simulink model "climateCtrl"  (Simulink 8.0)
settings: Solver=VariableStepDiscrete  StartTime=0.0  StopTime=20  RelTol=1e-3
PreLoadFcn:
  | dT = 2;
libraries: simulink x1
settings Model: Creator=jrivitus  LastModifiedBy=ZhouHaoyu
settings DataIOCC: SignalLoggingSaveFormat=ModelDataLogs
settings OptimizationCC: EfficientMapNaN2IntZero=off
settings DebuggingCC: FcnCallInpInsideContextMsg=UseLocalSettings  StrictBusMsg=Warning
settings GRTTargetCC: CombineOutputUpdateFcns=off  GRTInterface=on

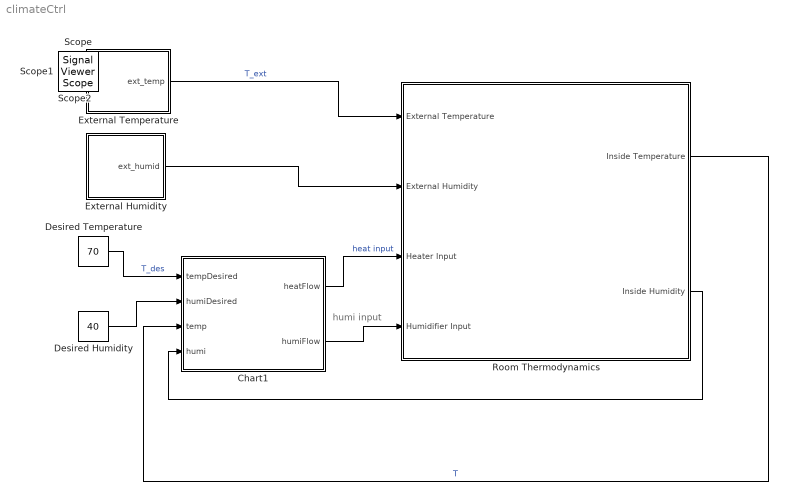
== system climateCtrl ==
  note: humi input
  Chart1 : Stateflow chart  TreatAsAtomicUnit=on
  Desired Humidity : Constant  Value=40
  Desired Temperature : Constant  Value=70
  External Humidity : Subsystem
  External Temperature : Subsystem
  Room Thermodynamics : Subsystem
  Scope : SignalViewerScope  IOType=viewer  RefreshTime=0.035000
      settings: TimeRange=20  YMin=50  YMax=100
  Scope1 : SignalViewerScope  IOType=viewer  RefreshTime=0.035000
  Scope2 : SignalViewerScope  IOType=viewer  RefreshTime=0.035000
      settings: SaveName=ScopeData2
  wires:
  External Temperature/1(ext_temp) -> Room Thermodynamics/1(External Temperature)  "T_ext"
  Chart1/1(heatFlow) -> Room Thermodynamics/3(Heater Input)  "heat input"
  Desired Temperature/1 -> Chart1/1(tempDesired)  "T_des"
  Room Thermodynamics/1(Inside Temperature) -> Chart1/3(temp)  "T"
  External Humidity/1(ext_humid) -> Room Thermodynamics/2(External Humidity)
  Room Thermodynamics/2(Inside Humidity) -> Chart1/4(humi)
  Desired Humidity/1 -> Chart1/2(humiDesired)
  Chart1/2(humiFlow) -> Room Thermodynamics/4(Humidifier Input)

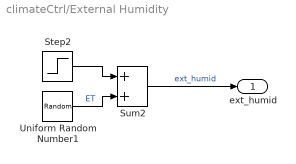
== system climateCtrl/External Humidity ==
  Step2 : Step  Time=10  Before=35  After=25  SampleTime=0.1
  Sum2 : Sum  SaturateOnIntegerOverflow=on
  Uniform Random Number1 : UniformRandomNumber  Minimum=-10  Maximum=10  SampleTime=0.1
  ext_humid : Outport
  wires:
  Sum2/1 -> ext_humid/1  "ext_humid"
  Step2/1 -> Sum2/1
  Uniform Random Number1/1 -> Sum2/2  "ET"

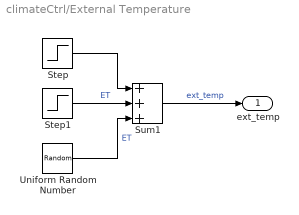
== system climateCtrl/External Temperature ==
  Step : Step  Time=15  Before=70  After=40  SampleTime=0.1
  Step1 : Step  Time=5  After=20  SampleTime=0.1
  Sum1 : Sum  Inputs=+++  SaturateOnIntegerOverflow=on
  Uniform Random Number : UniformRandomNumber  Minimum=-10  Maximum=10  SampleTime=0.1
  ext_temp : Outport
  wires:
  Step1/1 -> Sum1/2  "ET"
  Step/1 -> Sum1/1
  Uniform Random Number/1 -> Sum1/3  "ET"
  Sum1/1 -> ext_temp/1  "ext_temp"

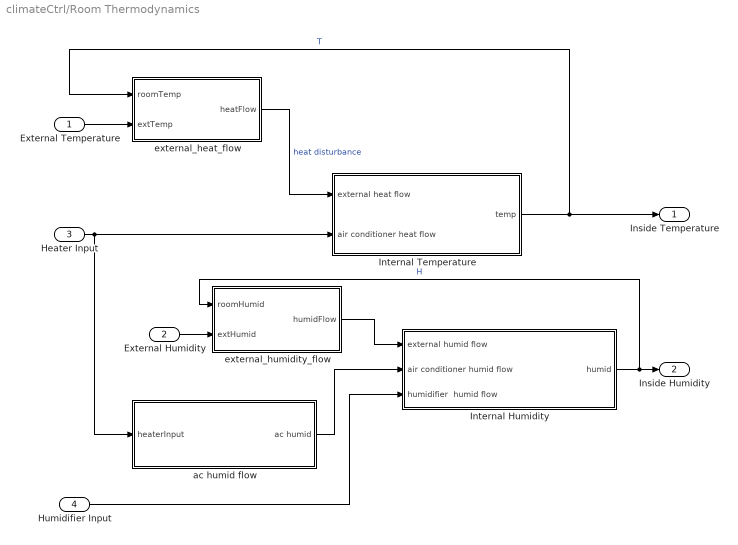
== system climateCtrl/Room Thermodynamics ==
  External Temperature : Inport
  External Humidity : Inport  Port=2
  Heater Input : Inport  Port=3
  Humidifier Input : Inport  Port=4
  Internal Humidity : Subsystem
  Internal Temperature : Subsystem
  ac humid flow : Subsystem
  external_heat_flow : Subsystem
  external_humidity_flow : Subsystem
  Inside Temperature : Outport
  Inside Humidity : Outport  Port=2
  wires:
  external_heat_flow/1(heatFlow) -> Internal Temperature/1(external heat flow)  "heat disturbance"
  Internal Temperature/1(temp) -> external_heat_flow/1(roomTemp), Inside Temperature/1  "T"
  External Temperature/1 -> external_heat_flow/2(extTemp)
  Heater Input/1 -> Internal Temperature/2(air conditioner heat flow), ac humid flow/1(heaterInput)
  External Humidity/1 -> external_humidity_flow/2(extHumid)
  external_humidity_flow/1(humidFlow) -> Internal Humidity/1(external humid flow)
  Internal Humidity/1(humid) -> external_humidity_flow/1(roomHumid), Inside Humidity/1  "H"
  Humidifier Input/1 -> Internal Humidity/3(humidifier  humid flow)
  ac humid flow/1(ac humid) -> Internal Humidity/2(air conditioner humid flow)

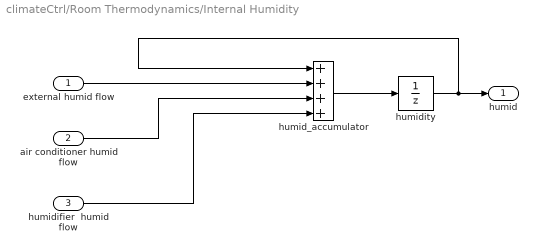
== system climateCtrl/Room Thermodynamics/Internal Humidity ==
  external humid flow : Inport
  air conditioner humid flow : Inport  Port=2
  humidifier  humid flow : Inport  Port=3
  humid_accumulator : Sum  Inputs=++++
  humidity : UnitDelay  InitialCondition=40  SampleTime=-1
  humid : Outport
  wires:
  air conditioner humid flow/1 -> humid_accumulator/3
  external humid flow/1 -> humid_accumulator/2
  humidity/1 -> humid_accumulator/1, humid/1
  humid_accumulator/1 -> humidity/1
  humidifier  humid flow/1 -> humid_accumulator/4

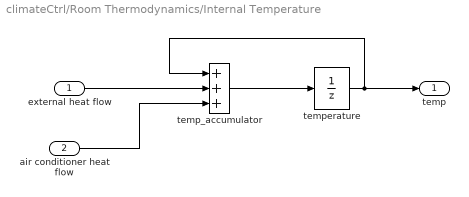
== system climateCtrl/Room Thermodynamics/Internal Temperature ==
  external heat flow : Inport
  air conditioner heat flow : Inport  Port=2
  temp_accumulator : Sum  Inputs=+++
  temperature : UnitDelay  InitialCondition=70  SampleTime=0.1
  temp : Outport
  wires:
  air conditioner heat flow/1 -> temp_accumulator/3
  external heat flow/1 -> temp_accumulator/2
  temp_accumulator/1 -> temperature/1
  temperature/1 -> temp/1, temp_accumulator/1

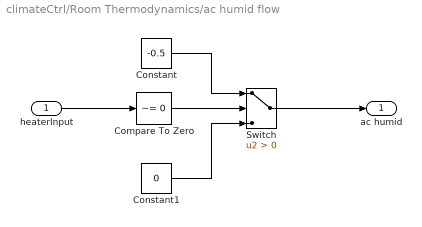
== system climateCtrl/Room Thermodynamics/ac humid flow ==
  heaterInput : Inport
  Compare To Zero : simulink/Logic and Bit Operations/Compare To Zero  relop=~=  OutDataTypeStr=uint8  ZeroCross=off
  Constant : Constant  Value=-0.5
  Constant1 : Constant  Value=0
  Switch : Switch  Criteria=u2 > Threshold
  ac humid : Outport  OutDataTypeStr=double  InitialOutput=0
  wires:
  heaterInput/1 -> Compare To Zero/1
  Compare To Zero/1 -> Switch/2
  Constant/1 -> Switch/1
  Constant1/1 -> Switch/3
  Switch/1 -> ac humid/1

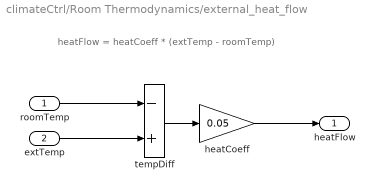
== system climateCtrl/Room Thermodynamics/external_heat_flow ==
  note: heatFlow = heatCoeff * (extTemp - roomTemp)
  roomTemp : Inport
  extTemp : Inport  Port=2
  heatCoeff : Gain  Gain=0.05
  tempDiff : Sum  Inputs=-+
  heatFlow : Outport  OutDataTypeStr=double  InitialOutput=0
  wires:
  extTemp/1 -> tempDiff/2
  roomTemp/1 -> tempDiff/1
  heatCoeff/1 -> heatFlow/1
  tempDiff/1 -> heatCoeff/1

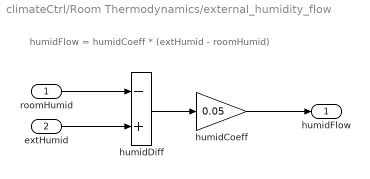
== system climateCtrl/Room Thermodynamics/external_humidity_flow ==
  note: humidFlow = humidCoeff * (extHumid - roomHumid)
  roomHumid : Inport
  extHumid : Inport  Port=2
  humidCoeff : Gain  Gain=0.05
  humidDiff : Sum  Inputs=-+
  humidFlow : Outport  OutDataTypeStr=double  InitialOutput=0
  wires:
  extHumid/1 -> humidDiff/2
  roomHumid/1 -> humidDiff/1
  humidDiff/1 -> humidCoeff/1
  humidCoeff/1 -> humidFlow/1

== stateflow chart Chart1 ==
  settings: executeAtInitialization=1
  state Off
    entry:
    heatFlow=0;
  state HeaterOn
    entry:
    heatFlow=1;
  state CoolerOn
    entry:
    heatFlow=-1;
  (default) -> Off
  Off -> HeaterOn [order 1] : [temp < (tempDesired-dT)]
  Off -> CoolerOn [order 2] : [temp > (tempDesired+dT)]
  CoolerOn -> Off [order 1] : [temp < (tempDesired+dT)]
  HeaterOn -> Off [order 1] : [temp > (tempDesired-dT)]
  HeaterOn -> HeaterOn [order 3] : [temp < (tempDesired-dT)&&humi>=humiDesired]{humiFlow=0;}
  CoolerOn -> CoolerOn [order 3] : [temp > (tempDesired+dT)&&humi>=humiDesired]{humiFlow=0;}
  CoolerOn -> CoolerOn [order 2] : [temp > (tempDesired+dT)&&humi<humiDesired]{humiFlow=1.5;}
  HeaterOn -> HeaterOn [order 2] : [temp < (tempDesired-dT)&&humi<humiDesired]{humiFlow=1.5;}
  data: tempDesired input double; humiDesired input double; heatFlow output double; temp input double; dT parameter double; humi input double; humiFlow output double
